simulink model "SubSistemaMecanico"  (R2023b)
settings: Solver=VariableStepAuto  StartTime=0.0  StopTime=10.0  RelTol=1e-3
values from neighbouring files (symbols this model uses):
  r = 120    [parametros_proyecto2.m]
undefined symbols (not defined in the file or in its folder): b_eq, k_l
settings Model: Creator=ignab  LastModifiedBy=ignab

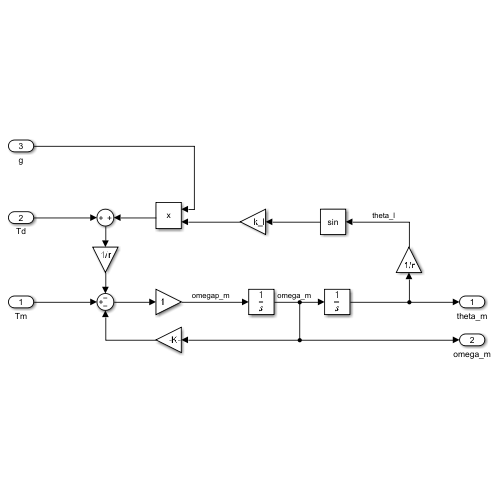
[thumbnail: Simulink's stored preview of the top-level diagram]
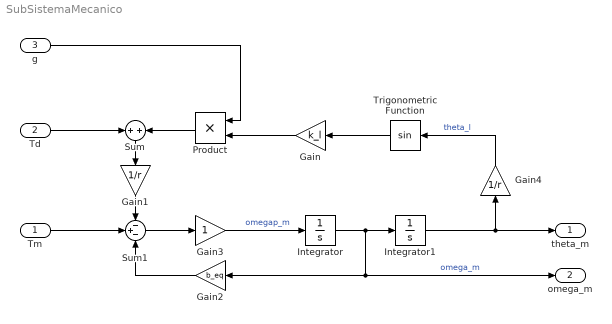
== system SubSistemaMecanico ==
  Tm : Inport
  Td : Inport  Port=2
  g : Inport  Port=3
  Gain : Gain  Gain=k_l
  Gain1 : Gain  Gain=1/r
  Gain2 : Gain  Gain=b_eq
  Gain3 : Gain
  Gain4 : Gain  Gain=1/r
  Integrator : Integrator
  Integrator1 : Integrator
  Product : Product
  Sum : Sum  Inputs=+|+
  Sum1 : Sum  Inputs=-+-
  Trigonometric Function : Trigonometry
  theta_m : Outport
  omega_m : Outport  Port=2
  wires:
  Td/1 -> Sum/1
  Product/1 -> Sum/2
  g/1 -> Product/1
  Gain/1 -> Product/2
  Sum/1 -> Gain1/1
  Gain1/1 -> Sum1/1
  Tm/1 -> Sum1/2
  Gain2/1 -> Sum1/3
  Sum1/1 -> Gain3/1
  Gain3/1 -> Integrator/1  "omegap_m"
  Integrator1/1 -> theta_m/1, Gain4/1
  Gain4/1 -> Trigonometric Function/1  "theta_l"
  Trigonometric Function/1 -> Gain/1
  Integrator/1 -> omega_m/1, Gain2/1, Integrator1/1  "omega_m"
